simulink model "QCar2_Virtual_Car2"  (R2023a)
settings: Solver=ode1  StartTime=0.0  StopTime=inf  FixedStep=cameraStepSize/10  RelTol=1e-3  EnableMultiTasking=on
PreLoadFcn:
  | QCarSetup
values from neighbouring files (symbols this model uses):
  cameraStepSize = 3e-2    (= 0.03)    [QCarSetup.m]
  path_x = [0.826 0.836 0.846 0.856 0.866 0.876 0.886 0.896 0.906 0.916 0.926 0.936 ... (740 elements, 740x1)]    [SDTS_Paths_6_2023.mat]
  path_x2 = [-0.614 -0.604 -0.594 -0.584 -0.574 -0.564 -0.554 -0.544 -0.534 -0.524 -0.514 -0.504 ... (1090 elements, 1090x1)]    [SDTS_Paths_6_2023.mat]
  path_x3 = [-0.614 -0.603821428571 -0.593642857143 -0.583464285714 -0.573285714286 -0.563107142857 -0.552928571429 -0.54275 -0.532571428571 -0.522392857143 -0.512214285714 -0.502035714286 ... (714 elements, 714x1)]    [SDTS_Paths_6_2023.mat]
  path_x4 = [-0.614 -0.604 -0.594 -0.584 -0.574 -0.564 -0.554 -0.544 -0.534 -0.524 -0.514 -0.504 ... (1761 elements, 1761x1)]    [SDTS_Paths_6_2023.mat]
  path_x5 = [1.436 1.42588571429 1.41577142857 1.40565714286 1.39554285714 1.38542857143 1.37531428571 1.3652 1.35508571429 1.34497142857 1.33485714286 1.32474285714 ... (574 elements, 574x1)]    [SDTS_Paths_6_2023.mat]
  path_x6 = [1.436 1.42588571429 1.41577142857 1.40565714286 1.39554285714 1.38542857143 1.37531428571 1.3652 1.35508571429 1.34497142857 1.33485714286 1.32474285714 ... (1288 elements, 1288x1)]    [SDTS_Paths_6_2023.mat]
  path_y = [-1.0887 -1.0887 -1.0887 -1.0887 -1.0887 -1.0887 -1.0887 -1.0887 -1.0887 -1.0887 -1.0887 -1.0887 ... (740 elements, 740x1)]    [SDTS_Paths_6_2023.mat]
  path_y2 = [-1.0887 -1.0887 -1.0887 -1.0887 -1.0887 -1.0887 -1.0887 -1.0887 -1.0887 -1.0887 -1.0887 -1.0887 ... (1090 elements, 1090x1)]    [SDTS_Paths_6_2023.mat]
  path_y3 = [-1.0887 -1.0887 -1.0887 -1.0887 -1.0887 -1.0887 -1.0887 -1.0887 -1.0887 -1.0887 -1.0887 -1.0887 ... (714 elements, 714x1)]    [SDTS_Paths_6_2023.mat]
  path_y4 = [-1.0887 -1.0887 -1.0887 -1.0887 -1.0887 -1.0887 -1.0887 -1.0887 -1.0887 -1.0887 -1.0887 -1.0887 ... (1761 elements, 1761x1)]    [SDTS_Paths_6_2023.mat]
  path_y5 = [-0.8157 -0.8157 -0.8157 -0.8157 -0.8157 -0.8157 -0.8157 -0.8157 -0.8157 -0.8157 -0.8157 -0.8157 ... (574 elements, 574x1)]    [SDTS_Paths_6_2023.mat]
  path_y6 = [-0.8157 -0.8157 -0.8157 -0.8157 -0.8157 -0.8157 -0.8157 -0.8157 -0.8157 -0.8157 -0.8157 -0.8157 ... (1288 elements, 1288x1)]    [SDTS_Paths_6_2023.mat]
undefined symbols (not defined in the file or in its folder): DiscIntNeverNeededParam, gcbh, height, Host, JPEG, left, qc_get_step_size, top, video_display_show, width
libraries: quarc_library x71, simulink_extras x12, simulink x5
(part 4 of 5)

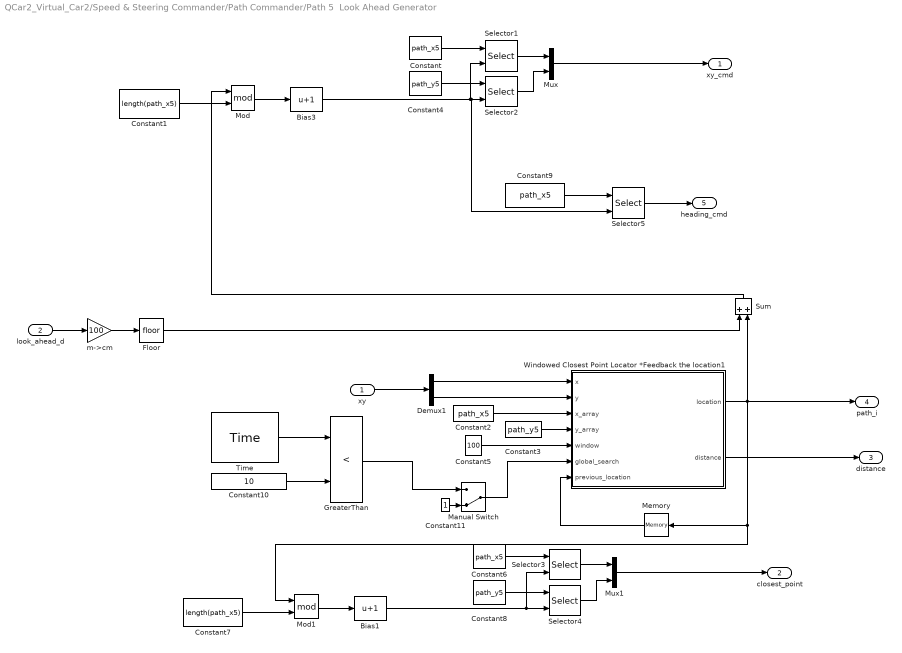
== system QCar2_Virtual_Car2/Speed & Steering Commander/Path Commander/Path 5  Look Ahead Generator ==
  xy : Inport
  look_ahead_d : Inport  Port=2
  Bias1 : Bias  Bias=1  SaturateOnIntegerOverflow=off
  Bias3 : Bias  Bias=1  SaturateOnIntegerOverflow=off
  Constant{,2,6,9} (4 alike) : Constant  Value=path_x5
  Constant1 : Constant  Value=length(path_x5)
  Constant10 : Constant  Value=10
  Constant11 : Constant
  Constant3 : Constant  Value=path_y5
  Constant4 : Constant  Value=path_y5
  Constant5 : Constant  Value=100
  Constant7 : Constant  Value=length(path_x5)
  Constant8 : Constant  Value=path_y5
  Demux1 : Demux  Outputs=2
  Floor : Rounding
  GreaterThan : RelationalOperator  Operator=<  OutDataTypeStr=boolean  RndMeth=Simplest  InputSameDT=off
  Manual Switch : ManualSwitch  CurrentSetting=0
  Memory : Memory  InitialCondition=1  InheritSampleTime=on  LinearizeMemory=on  LinearizeAsDelay=on
  Mod : Math  Operator=mod
  Mod1 : Math  Operator=mod
  Mux : Mux  Inputs=2
  Mux1 : Mux  Inputs=2
  Selector{1..5} (5 alike) : Selector  InputPortWidth=length(path_x5)  IndexOptions=Index vector (port)  Indices=[1 3]  OutputSizes=1
  Sum : Sum
  Time : quarc_library/Sources/Time/Time  time_source=Wall clock  sample_time=qc_get_step_size
  Windowed Closest Point Locator *Feedback the location1 : MATLAB Function  TreatAsAtomicUnit=on
  m->cm : Gain  Gain=100
  xy_cmd : Outport
  closest_point : Outport  Port=2
  distance : Outport  Port=3
  path_i : Outport  Port=4
  heading_cmd : Outport  Port=5
  wires:
  Windowed Closest Point Locator *Feedback the location1/1(location) -> Mod1/1, Memory/1, path_i/1, Sum/2
  Memory/1 -> Windowed Closest Point Locator *Feedback the location1/7(previous_location)
  Constant5/1 -> Windowed Closest Point Locator *Feedback the location1/5(window)
  Selector5/1 -> heading_cmd/1
  Constant9/1 -> Selector5/1
  Bias3/1 -> Selector2/2, Selector5/2, Selector1/2
  Windowed Closest Point Locator *Feedback the location1/2(distance) -> distance/1
  Selector2/1 -> Mux/2
  Mux/1 -> xy_cmd/1
  Constant4/1 -> Selector2/1
  Selector1/1 -> Mux/1
  Constant/1 -> Selector1/1
  Floor/1 -> Sum/1
  m->cm/1 -> Floor/1
  look_ahead_d/1 -> m->cm/1
  xy/1 -> Demux1/1
  Mod/1 -> Bias3/1
  Demux1/2 -> Windowed Closest Point Locator *Feedback the location1/2(y)
  Sum/1 -> Mod/1
  Constant1/1 -> Mod/2
  Constant3/1 -> Windowed Closest Point Locator *Feedback the location1/4(y_array)
  Constant2/1 -> Windowed Closest Point Locator *Feedback the location1/3(x_array)
  Demux1/1 -> Windowed Closest Point Locator *Feedback the location1/1(x)
  Mux1/1 -> closest_point/1
  Mod1/1 -> Bias1/1
  Selector4/1 -> Mux1/2
  Constant7/1 -> Mod1/2
  Selector3/1 -> Mux1/1
  Constant8/1 -> Selector4/1
  Bias1/1 -> Selector3/2, Selector4/2
  Constant6/1 -> Selector3/1
  Time/1 -> GreaterThan/1
  Constant10/1 -> GreaterThan/2
  Manual Switch/1 -> Windowed Closest Point Locator *Feedback the location1/6(global_search)
  Constant11/1 -> Manual Switch/2
  GreaterThan/1 -> Manual Switch/1

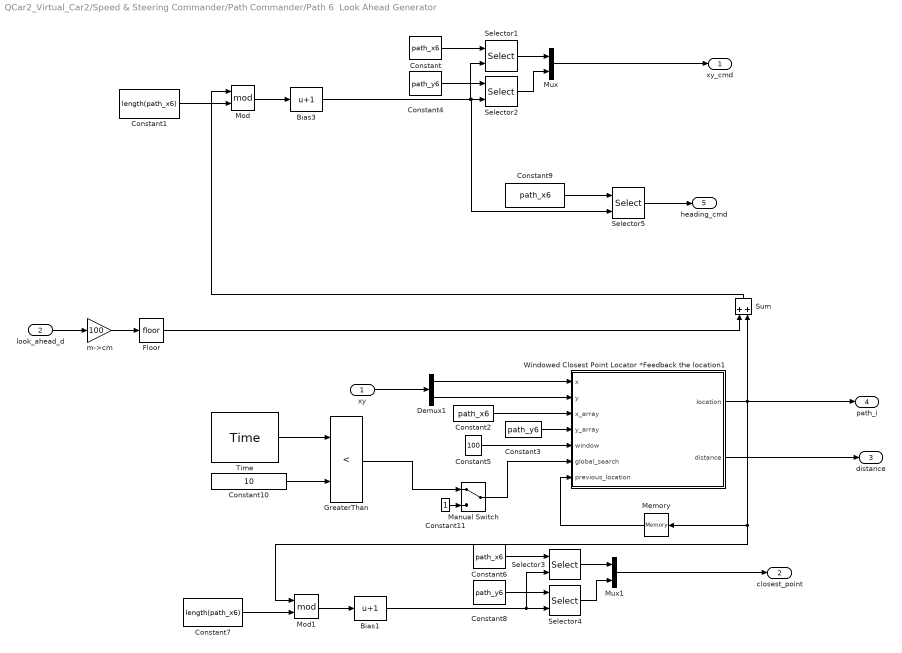
== system QCar2_Virtual_Car2/Speed & Steering Commander/Path Commander/Path 6  Look Ahead Generator ==
  xy : Inport
  look_ahead_d : Inport  Port=2
  Bias1 : Bias  Bias=1  SaturateOnIntegerOverflow=off
  Bias3 : Bias  Bias=1  SaturateOnIntegerOverflow=off
  Constant{,2,6,9} (4 alike) : Constant  Value=path_x6
  Constant1 : Constant  Value=length(path_x6)
  Constant10 : Constant  Value=10
  Constant11 : Constant
  Constant3 : Constant  Value=path_y6
  Constant4 : Constant  Value=path_y6
  Constant5 : Constant  Value=100
  Constant7 : Constant  Value=length(path_x6)
  Constant8 : Constant  Value=path_y6
  Demux1 : Demux  Outputs=2
  Floor : Rounding
  GreaterThan : RelationalOperator  Operator=<  OutDataTypeStr=boolean  RndMeth=Simplest  InputSameDT=off
  Manual Switch : ManualSwitch
  Memory : Memory  InitialCondition=1  InheritSampleTime=on  LinearizeMemory=on  LinearizeAsDelay=on
  Mod : Math  Operator=mod
  Mod1 : Math  Operator=mod
  Mux : Mux  Inputs=2
  Mux1 : Mux  Inputs=2
  Selector{1..5} (5 alike) : Selector  InputPortWidth=length(path_x6)  IndexOptions=Index vector (port)  Indices=[1 3]  OutputSizes=1
  Sum : Sum
  Time : quarc_library/Sources/Time/Time  time_source=Wall clock  sample_time=qc_get_step_size
  Windowed Closest Point Locator *Feedback the location1 : MATLAB Function  TreatAsAtomicUnit=on
  m->cm : Gain  Gain=100
  xy_cmd : Outport
  closest_point : Outport  Port=2
  distance : Outport  Port=3
  path_i : Outport  Port=4
  heading_cmd : Outport  Port=5
  wires:
  GreaterThan/1 -> Manual Switch/1
  Constant11/1 -> Manual Switch/2
  Manual Switch/1 -> Windowed Closest Point Locator *Feedback the location1/6(global_search)
  Constant10/1 -> GreaterThan/2
  Time/1 -> GreaterThan/1
  Constant6/1 -> Selector3/1
  Bias1/1 -> Selector4/2, Selector3/2
  Constant8/1 -> Selector4/1
  Selector3/1 -> Mux1/1
  Constant7/1 -> Mod1/2
  Selector4/1 -> Mux1/2
  Mod1/1 -> Bias1/1
  Mux1/1 -> closest_point/1
  Demux1/1 -> Windowed Closest Point Locator *Feedback the location1/1(x)
  Constant2/1 -> Windowed Closest Point Locator *Feedback the location1/3(x_array)
  Constant3/1 -> Windowed Closest Point Locator *Feedback the location1/4(y_array)
  Constant1/1 -> Mod/2
  Sum/1 -> Mod/1
  Demux1/2 -> Windowed Closest Point Locator *Feedback the location1/2(y)
  Mod/1 -> Bias3/1
  xy/1 -> Demux1/1
  look_ahead_d/1 -> m->cm/1
  m->cm/1 -> Floor/1
  Floor/1 -> Sum/1
  Constant/1 -> Selector1/1
  Selector1/1 -> Mux/1
  Constant4/1 -> Selector2/1
  Mux/1 -> xy_cmd/1
  Selector2/1 -> Mux/2
  Windowed Closest Point Locator *Feedback the location1/2(distance) -> distance/1
  Bias3/1 -> Selector1/2, Selector5/2, Selector2/2
  Constant9/1 -> Selector5/1
  Selector5/1 -> heading_cmd/1
  Constant5/1 -> Windowed Closest Point Locator *Feedback the location1/5(window)
  Memory/1 -> Windowed Closest Point Locator *Feedback the location1/7(previous_location)
  Windowed Closest Point Locator *Feedback the location1/1(location) -> Sum/2, path_i/1, Memory/1, Mod1/1

== system QCar2_Virtual_Car2/Speed & Steering Commander/Traffic Zone 1/Greater Than Threshold ==
  Signal : Inport
  Threshold : Inport  Port=2
  Duration : Inport  Port=3
  Data Type Conversion : DataTypeConversion  SaturateOnIntegerOverflow=off  RndMeth=Floor
  Discrete-Time Integrator : DiscreteIntegrator  Priority=1  ExternalReset=level  SampleTime=qc_get_step_size  ICPrevOutput=DiscIntNeverNeededParam  ICPrevScaledInput=DiscIntNeverNeededParam
  Logical Operator : Logic  Operator=NOT  AllPortsSameDT=off  OutDataTypeStr=boolean
  Relational Operator : RelationalOperator  InputSameDT=off
  Relational Operator1 : RelationalOperator  InputSameDT=off
  elapsed : Outport  VectorParamsAs1DForOutWhenUnconnected=off
  time : Outport  Port=2  VectorParamsAs1DForOutWhenUnconnected=off
  wires:
  Relational Operator1/1 -> elapsed/1
  Duration/1 -> Relational Operator1/2
  Discrete-Time Integrator/1 -> time/1, Relational Operator1/1
  Logical Operator/1 -> Discrete-Time Integrator/2
  Relational Operator/1 -> Logical Operator/1, Data Type Conversion/1
  Threshold/1 -> Relational Operator/2
  Signal/1 -> Relational Operator/1
  Data Type Conversion/1 -> Discrete-Time Integrator/1

== system QCar2_Virtual_Car2/Speed & Steering Commander/Traffic Zone 1/Less Than Threshold ==
  Signal : Inport
  Threshold : Inport  Port=2
  Duration : Inport  Port=3
  Data Type Conversion : DataTypeConversion  SaturateOnIntegerOverflow=off  RndMeth=Floor
  Discrete-Time Integrator : DiscreteIntegrator  Priority=1  ExternalReset=level  SampleTime=qc_get_step_size  ICPrevOutput=DiscIntNeverNeededParam  ICPrevScaledInput=DiscIntNeverNeededParam
  Logical Operator : Logic  Operator=NOT  AllPortsSameDT=off  OutDataTypeStr=boolean
  Relational Operator : RelationalOperator  Operator=<  InputSameDT=off
  Relational Operator1 : RelationalOperator  InputSameDT=off
  elapsed : Outport  VectorParamsAs1DForOutWhenUnconnected=off
  time : Outport  Port=2  VectorParamsAs1DForOutWhenUnconnected=off
  wires:
  Data Type Conversion/1 -> Discrete-Time Integrator/1
  Signal/1 -> Relational Operator/1
  Threshold/1 -> Relational Operator/2
  Relational Operator/1 -> Data Type Conversion/1, Logical Operator/1
  Logical Operator/1 -> Discrete-Time Integrator/2
  Discrete-Time Integrator/1 -> Relational Operator1/1, time/1
  Duration/1 -> Relational Operator1/2
  Relational Operator1/1 -> elapsed/1

== system QCar2_Virtual_Car2/Speed & Steering Commander/Traffic Zone 2/Greater Than Threshold ==
  Signal : Inport
  Threshold : Inport  Port=2
  Duration : Inport  Port=3
  Data Type Conversion : DataTypeConversion  SaturateOnIntegerOverflow=off  RndMeth=Floor
  Discrete-Time Integrator : DiscreteIntegrator  Priority=1  ExternalReset=level  SampleTime=qc_get_step_size  ICPrevOutput=DiscIntNeverNeededParam  ICPrevScaledInput=DiscIntNeverNeededParam
  Logical Operator : Logic  Operator=NOT  AllPortsSameDT=off  OutDataTypeStr=boolean
  Relational Operator : RelationalOperator  InputSameDT=off
  Relational Operator1 : RelationalOperator  InputSameDT=off
  elapsed : Outport  VectorParamsAs1DForOutWhenUnconnected=off
  time : Outport  Port=2  VectorParamsAs1DForOutWhenUnconnected=off
  wires:
  Data Type Conversion/1 -> Discrete-Time Integrator/1
  Signal/1 -> Relational Operator/1
  Threshold/1 -> Relational Operator/2
  Relational Operator/1 -> Data Type Conversion/1, Logical Operator/1
  Logical Operator/1 -> Discrete-Time Integrator/2
  Discrete-Time Integrator/1 -> Relational Operator1/1, time/1
  Duration/1 -> Relational Operator1/2
  Relational Operator1/1 -> elapsed/1

== system QCar2_Virtual_Car2/Speed & Steering Commander/Traffic Zone 2/Less Than Threshold ==
  Signal : Inport
  Threshold : Inport  Port=2
  Duration : Inport  Port=3
  Data Type Conversion : DataTypeConversion  SaturateOnIntegerOverflow=off  RndMeth=Floor
  Discrete-Time Integrator : DiscreteIntegrator  Priority=1  ExternalReset=level  SampleTime=qc_get_step_size  ICPrevOutput=DiscIntNeverNeededParam  ICPrevScaledInput=DiscIntNeverNeededParam
  Logical Operator : Logic  Operator=NOT  AllPortsSameDT=off  OutDataTypeStr=boolean
  Relational Operator : RelationalOperator  Operator=<  InputSameDT=off
  Relational Operator1 : RelationalOperator  InputSameDT=off
  elapsed : Outport  VectorParamsAs1DForOutWhenUnconnected=off
  time : Outport  Port=2  VectorParamsAs1DForOutWhenUnconnected=off
  wires:
  Relational Operator1/1 -> elapsed/1
  Duration/1 -> Relational Operator1/2
  Discrete-Time Integrator/1 -> time/1, Relational Operator1/1
  Logical Operator/1 -> Discrete-Time Integrator/2
  Relational Operator/1 -> Logical Operator/1, Data Type Conversion/1
  Threshold/1 -> Relational Operator/2
  Signal/1 -> Relational Operator/1
  Data Type Conversion/1 -> Discrete-Time Integrator/1

== system QCar2_Virtual_Car2/Cameras/CSI Camera/Extract Center and Slope/Angle Check ==
  score : Inport
  Angle In : Inport  Port=2
  score threshold : Inport  Port=3
  IsNaN : RelationalOperator  Operator=isNaN  OutDataTypeStr=boolean  RndMeth=Simplest  InputSameDT=off
  Less Than : RelationalOperator  Operator=<  OutDataTypeStr=boolean  RndMeth=Simplest  InputSameDT=off
  MATLAB Function1 : MATLAB Function  TreatAsAtomicUnit=on
  Memory : Memory  InheritSampleTime=on  LinearizeMemory=on  LinearizeAsDelay=on
  OR : Logic  Operator=OR  IconShape=distinctive  AllPortsSameDT=off  OutDataTypeStr=boolean
  Angle Out : Outport  VectorParamsAs1DForOutWhenUnconnected=off
  wires:
  IsNaN/1 -> OR/1
  OR/1 -> MATLAB Function1/2(is_nan)
  Less Than/1 -> OR/2
  score/1 -> Less Than/1
  score threshold/1 -> Less Than/2
  MATLAB Function1/1(output) -> Angle Out/1, Memory/1
  Angle In/1 -> MATLAB Function1/1(input), IsNaN/1
  Memory/1 -> MATLAB Function1/3(prev_output)

== system QCar2_Virtual_Car2/Cameras/CSI Camera/Extract Center and Slope/Center Check ==
  score : Inport
  Center : Inport  Port=2
  score threshold : Inport  Port=3
  IsNaN : RelationalOperator  Operator=isNaN  OutDataTypeStr=boolean  RndMeth=Simplest  InputSameDT=off
  Less Than : RelationalOperator  Operator=<  OutDataTypeStr=boolean  RndMeth=Simplest  InputSameDT=off
  MATLAB Function1 : MATLAB Function  TreatAsAtomicUnit=on
  Memory : Memory  InitialCondition=640/2  InheritSampleTime=on  LinearizeMemory=on  LinearizeAsDelay=on
  OR : Logic  Operator=OR  IconShape=distinctive  AllPortsSameDT=off  OutDataTypeStr=boolean
  Center Out : Outport  VectorParamsAs1DForOutWhenUnconnected=off
  wires:
  score threshold/1 -> Less Than/2
  Less Than/1 -> OR/2
  score/1 -> Less Than/1
  IsNaN/1 -> OR/1
  OR/1 -> MATLAB Function1/2(is_nan)
  Memory/1 -> MATLAB Function1/3(prev_output)
  Center/1 -> IsNaN/1, MATLAB Function1/1(input)
  MATLAB Function1/1(output) -> Memory/1, Center Out/1

== system QCar2_Virtual_Car2/QCar/Virtual QCar/LED Logic/Greater Than Threshold1 ==
  Signal : Inport
  Threshold : Inport  Port=2
  Duration : Inport  Port=3
  Data Type Conversion : DataTypeConversion  SaturateOnIntegerOverflow=off  RndMeth=Floor
  Discrete-Time Integrator : DiscreteIntegrator  Priority=1  ExternalReset=level  SampleTime=qc_get_step_size  ICPrevOutput=DiscIntNeverNeededParam  ICPrevScaledInput=DiscIntNeverNeededParam
  Logical Operator : Logic  Operator=NOT  AllPortsSameDT=off  OutDataTypeStr=boolean
  Relational Operator : RelationalOperator  InputSameDT=off
  Relational Operator1 : RelationalOperator  InputSameDT=off
  elapsed : Outport  VectorParamsAs1DForOutWhenUnconnected=off
  time : Outport  Port=2  VectorParamsAs1DForOutWhenUnconnected=off
  wires:
  Data Type Conversion/1 -> Discrete-Time Integrator/1
  Signal/1 -> Relational Operator/1
  Threshold/1 -> Relational Operator/2
  Relational Operator/1 -> Data Type Conversion/1, Logical Operator/1
  Logical Operator/1 -> Discrete-Time Integrator/2
  Discrete-Time Integrator/1 -> Relational Operator1/1, time/1
  Duration/1 -> Relational Operator1/2
  Relational Operator1/1 -> elapsed/1

== system QCar2_Virtual_Car2/QCar/Virtual QCar/LED Logic/Left Threshold ==
  Signal : Inport
  Threshold : Inport  Port=2
  Duration : Inport  Port=3
  Data Type Conversion : DataTypeConversion  SaturateOnIntegerOverflow=off  RndMeth=Floor
  Discrete-Time Integrator : DiscreteIntegrator  Priority=1  ExternalReset=level  SampleTime=qc_get_step_size  ICPrevOutput=DiscIntNeverNeededParam  ICPrevScaledInput=DiscIntNeverNeededParam
  Logical Operator : Logic  Operator=NOT  AllPortsSameDT=off  OutDataTypeStr=boolean
  Relational Operator : RelationalOperator  InputSameDT=off
  Relational Operator1 : RelationalOperator  InputSameDT=off
  elapsed : Outport  VectorParamsAs1DForOutWhenUnconnected=off
  time : Outport  Port=2  VectorParamsAs1DForOutWhenUnconnected=off
  wires:
  Data Type Conversion/1 -> Discrete-Time Integrator/1
  Signal/1 -> Relational Operator/1
  Threshold/1 -> Relational Operator/2
  Relational Operator/1 -> Data Type Conversion/1, Logical Operator/1
  Logical Operator/1 -> Discrete-Time Integrator/2
  Discrete-Time Integrator/1 -> Relational Operator1/1, time/1
  Duration/1 -> Relational Operator1/2
  Relational Operator1/1 -> elapsed/1

== system QCar2_Virtual_Car2/QCar/Virtual QCar/LED Logic/Less Than Threshold1 ==
  Signal : Inport
  Threshold : Inport  Port=2
  Duration : Inport  Port=3
  Data Type Conversion : DataTypeConversion  SaturateOnIntegerOverflow=off  RndMeth=Floor
  Discrete-Time Integrator : DiscreteIntegrator  Priority=1  ExternalReset=level  SampleTime=qc_get_step_size  ICPrevOutput=DiscIntNeverNeededParam  ICPrevScaledInput=DiscIntNeverNeededParam
  Logical Operator : Logic  Operator=NOT  AllPortsSameDT=off  OutDataTypeStr=boolean
  Relational Operator : RelationalOperator  Operator=<  InputSameDT=off
  Relational Operator1 : RelationalOperator  InputSameDT=off
  elapsed : Outport  VectorParamsAs1DForOutWhenUnconnected=off
  time : Outport  Port=2  VectorParamsAs1DForOutWhenUnconnected=off
  wires:
  Relational Operator1/1 -> elapsed/1
  Duration/1 -> Relational Operator1/2
  Discrete-Time Integrator/1 -> time/1, Relational Operator1/1
  Logical Operator/1 -> Discrete-Time Integrator/2
  Relational Operator/1 -> Logical Operator/1, Data Type Conversion/1
  Threshold/1 -> Relational Operator/2
  Signal/1 -> Relational Operator/1
  Data Type Conversion/1 -> Discrete-Time Integrator/1

== system QCar2_Virtual_Car2/QCar/Virtual QCar/LED Logic/Less Than Threshold2 ==
  Signal : Inport
  Threshold : Inport  Port=2
  Duration : Inport  Port=3
  Data Type Conversion : DataTypeConversion  SaturateOnIntegerOverflow=off  RndMeth=Floor
  Discrete-Time Integrator : DiscreteIntegrator  Priority=1  ExternalReset=level  SampleTime=qc_get_step_size  ICPrevOutput=DiscIntNeverNeededParam  ICPrevScaledInput=DiscIntNeverNeededParam
  Logical Operator : Logic  Operator=NOT  AllPortsSameDT=off  OutDataTypeStr=boolean
  Relational Operator : RelationalOperator  Operator=<  InputSameDT=off
  Relational Operator1 : RelationalOperator  InputSameDT=off
  elapsed : Outport  VectorParamsAs1DForOutWhenUnconnected=off
  time : Outport  Port=2  VectorParamsAs1DForOutWhenUnconnected=off
  wires:
  Data Type Conversion/1 -> Discrete-Time Integrator/1
  Signal/1 -> Relational Operator/1
  Threshold/1 -> Relational Operator/2
  Relational Operator/1 -> Data Type Conversion/1, Logical Operator/1
  Logical Operator/1 -> Discrete-Time Integrator/2
  Discrete-Time Integrator/1 -> Relational Operator1/1, time/1
  Duration/1 -> Relational Operator1/2
  Relational Operator1/1 -> elapsed/1

== system QCar2_Virtual_Car2/QCar/Virtual QCar/LED Logic/Less Than Threshold3 ==
  Signal : Inport
  Threshold : Inport  Port=2
  Duration : Inport  Port=3
  Data Type Conversion : DataTypeConversion  SaturateOnIntegerOverflow=off  RndMeth=Floor
  Discrete-Time Integrator : DiscreteIntegrator  Priority=1  ExternalReset=level  SampleTime=qc_get_step_size  ICPrevOutput=DiscIntNeverNeededParam  ICPrevScaledInput=DiscIntNeverNeededParam
  Logical Operator : Logic  Operator=NOT  AllPortsSameDT=off  OutDataTypeStr=boolean
  Relational Operator : RelationalOperator  Operator=<  InputSameDT=off
  Relational Operator1 : RelationalOperator  InputSameDT=off
  elapsed : Outport  VectorParamsAs1DForOutWhenUnconnected=off
  time : Outport  Port=2  VectorParamsAs1DForOutWhenUnconnected=off
  wires:
  Relational Operator1/1 -> elapsed/1
  Duration/1 -> Relational Operator1/2
  Discrete-Time Integrator/1 -> time/1, Relational Operator1/1
  Logical Operator/1 -> Discrete-Time Integrator/2
  Relational Operator/1 -> Logical Operator/1, Data Type Conversion/1
  Threshold/1 -> Relational Operator/2
  Signal/1 -> Relational Operator/1
  Data Type Conversion/1 -> Discrete-Time Integrator/1

== system QCar2_Virtual_Car2/QCar/Virtual QCar/LED Logic/Right Threshold ==
  Signal : Inport
  Threshold : Inport  Port=2
  Duration : Inport  Port=3
  Data Type Conversion : DataTypeConversion  SaturateOnIntegerOverflow=off  RndMeth=Floor
  Discrete-Time Integrator : DiscreteIntegrator  Priority=1  ExternalReset=level  SampleTime=qc_get_step_size  ICPrevOutput=DiscIntNeverNeededParam  ICPrevScaledInput=DiscIntNeverNeededParam
  Logical Operator : Logic  Operator=NOT  AllPortsSameDT=off  OutDataTypeStr=boolean
  Relational Operator : RelationalOperator  Operator=<  InputSameDT=off
  Relational Operator1 : RelationalOperator  InputSameDT=off
  elapsed : Outport  VectorParamsAs1DForOutWhenUnconnected=off
  time : Outport  Port=2  VectorParamsAs1DForOutWhenUnconnected=off
  wires:
  Data Type Conversion/1 -> Discrete-Time Integrator/1
  Signal/1 -> Relational Operator/1
  Threshold/1 -> Relational Operator/2
  Relational Operator/1 -> Data Type Conversion/1, Logical Operator/1
  Logical Operator/1 -> Discrete-Time Integrator/2
  Discrete-Time Integrator/1 -> Relational Operator1/1, time/1
  Duration/1 -> Relational Operator1/2
  Relational Operator1/1 -> elapsed/1

== matlab function QCar2_Virtual_Car2/Speed & Steering Commander/Traffic Zone 2/MATLAB Function2 ==
  data: Previous_State input; Speed_In input; Speed_Multi input; In_Zone input; Traffic_State output; Speed_Out output; Traffic_Light input
function [Traffic_State, Speed_Out]  = Traffic_Controller (Previous_State, Speed_In, Speed_Multi, In_Zone, Traffic_Light)
%#codegen
Traffic_State = Previous_State;
Speed_Out = Speed_In;

switch Traffic_State
    % Case 1 - Normal - either not in zone or green light, Case 2 - red
    % light and in zone
    
    case 1
        % Green light or not in zone
        Speed_Out = Speed_In;
        if (Traffic_Light == 0) && (In_Zone == 1)
            % Caught in the traffic controller's web!
            Traffic_State = 2;
        end
        
    case 2
        % Red light state
        Speed_Out = Speed_In * Speed_Multi;
        
        if (Traffic_Light == 1)
            % Green Light
            Traffic_State = 1;
        end
        
end
end

== matlab function QCar2_Virtual_Car2/QCar/To//From Simulation/Receive Fcn ==
  data: Receive input size=800000; RequestServerUpdate output; New input; Location output; Rotation output; BumpForward output; BumpRear output; EnvironmentReset output; LidarDist output; LidarAngle output; NewCSIRight output; ImageCSIRight output size=100000; NewCSIRear output; ImageCSIRear output size=100000; NewCSILeft output; ImageCSILeft output size=100000; NewCSIFront output; ImageCSIFront output size=100000; NewRGB output; ImageRGB output size=100000; NewDepth output; ImageDepth output size=100000; Debug output
function [RequestServerUpdate, Location, Rotation, BumpForward, BumpRear, EnvironmentReset, LidarDist, LidarAngle, ...
    NewCSIRight, ImageCSIRight, ...
    NewCSIRear, ImageCSIRear, ...
    NewCSILeft, ImageCSILeft, ...
    NewCSIFront, ImageCSIFront, ...
    NewRGB, ImageRGB, ...
    NewDepth, ImageDepth, ...
    Debug]  = QCar2ApplicationWorkspaceDecodeDataPacket(Receive, New)

%% Setup

LIDAR_SAMPLES = 384;
LIDAR_RANGE = 80;

persistent iLocation;
persistent iRotation;
persistent iBumpForward;
persistent iBumpRear;
persistent iLidarDist;
persistent iLidarAngle;

if isempty(iLocation)
    iLocation = [single(0); single(0); single(0)];
    iRotation = [single(0); single(0); single(0)];
    iBumpForward = uint8(0);
    iBumpRear = uint8(0);
    iLidarAngle = zeros(1,LIDAR_SAMPLES);   
    iLidarDist = zeros(1,LIDAR_SAMPLES);      
end

% Need to assign outputs here even though they are reassigned at the end
% since matlab can't determine the signal widths
Location = [single(0); single(0); single(0)];
Rotation = [single(0); single(0); single(0)];
BumpForward = uint8(0);
BumpRear = uint8(0);
EnvironmentReset = 0;

LidarAngle = zeros(1,LIDAR_SAMPLES);
LidarDist = zeros(1,LIDAR_SAMPLES);

ImageCSIRight = uint8([]);
NewCSIRight = 0;
ImageCSIRear = uint8([]);
NewCSIRear = 0;
ImageCSILeft = uint8([]);
NewCSILeft = 0;
ImageCSIFront = uint8([]);
NewCSIFront = 0;
ImageRGB = uint8([]);
NewRGB = 0;
ImageDepth = uint8([]);
NewDepth = 0;


RequestServerUpdate = uint8(0);
PacketSize = length(Receive);

Debug = int32(0);

% Packet > 0, new data, and magic number in first index
if ((PacketSize > 0) && (New == 1) && (Receive(1) == uint8(123)))
    
    %skip magic number
    Index = int32(2);
    
    while(Index <= PacketSize)
       
        %% Get container details
        ContainerSize = typecast(uint8(flip(Receive(Index:Index+3))), 'int32');
        DeviceID = typecast(uint8(flip(Receive(Index+4:Index+7))), 'int32');
        DeviceNum = typecast(uint8(flip(Receive(Index+8:Index+11))), 'int32');
        DeviceFunction = uint8(Receive(Index+12));
        PayloadStart = Index+13;
        PayloadEnd = Index+ContainerSize-1;
        
        %% Pass container to appropriate decoding function
        if (DeviceID == 161) %is this a QCar 2 container?
            
            if (DeviceFunction == 11) %UE4 State Response
                [iLocation, iRotation, iBumpForward, iBumpRear] = QCar2DecodeVelocityStateContainer(Receive, PayloadStart);
                RequestServerUpdate = uint8(11);
            elseif (DeviceFunction == 101) % Pull out RGB payload for external processing
                CameraNum = typecast(uint8(flip(Receive(PayloadStart:PayloadStart+3))), 'int32');
                ImageSize = typecast(uint8(flip(Receive(PayloadStart+4:PayloadStart+7))), 'int32');
                
                if CameraNum == 0
                    ImageCSIRight = Receive(PayloadStart+8:PayloadEnd);
                    NewCSIRight = 1;
                    
                elseif CameraNum == 1
                    ImageCSIRear = Receive(PayloadStart+8:PayloadEnd);
                    NewCSIRear = 1;
                    
                elseif CameraNum == 2
                    ImageCSILeft = Receive(PayloadStart+8:PayloadEnd);
                    NewCSILeft = 1;
                    
                elseif CameraNum == 3
                    ImageCSIFront = Receive(PayloadStart+8:PayloadEnd);
                    NewCSIFront = 1;
                    
                elseif CameraNum == 4
                    ImageRGB = Receive(PayloadStart+8:PayloadEnd);
                    NewRGB = 1;
                    
                elseif CameraNum == 5
                    ImageDepth = Receive(PayloadStart+8:PayloadEnd);
                    NewDepth = 1;
                end
                RequestServerUpdate = uint8(1);

            elseif (DeviceFunction == 111) % Process LIDAR
                [iLidarAngle, iLidarDist] = QCar2DecodeLidarContainer(Receive, PayloadStart, LIDAR_SAMPLES, LIDAR_RANGE);
                RequestServerUpdate = uint8(1);                
            end
        elseif (DeviceID == 1001) %Simulink notification
            if (DeviceFunction == 200) %Reset button
                EnvironmentReset = 1;
            end
            


        end
       
        
        %% Process next container if any data is left.
        Index = Index+ContainerSize;
    end


end

Location = iLocation;
Rotation = iRotation;
BumpForward = iBumpForward;
BumpRear = iBumpRear;
LidarDist = iLidarDist;
LidarAngle = iLidarAngle;

== matlab function QCar2_Virtual_Car2/Speed & Steering Commander/Adaptive Cruise Control/MATLAB Function ==
  data: obstacle_distance input; speed_cmd output; stop_distance input; nominal_tracking_distance input; nominal_speed input
function speed_cmd = adaptive_cruise_control(obstacle_distance, stop_distance, nominal_tracking_distance, nominal_speed)

speed_cmd = nominal_speed;

if obstacle_distance < stop_distance
    speed_cmd = sat(nominal_speed,0,-1);
    
elseif obstacle_distance < nominal_tracking_distance
    speed_cmd = nominal_speed/(nominal_tracking_distance-stop_distance)*obstacle_distance - nominal_speed/(nominal_tracking_distance-stop_distance)*stop_distance;
end

function output = sat (input, max,min)
if input > max
    output = max;
elseif input < min
    output = min;
else
    output = input;
end

== matlab function QCar2_Virtual_Car2/Speed & Steering Commander/LiDAR Steering/Steering Commander ==
  data: steering output; aoa input
function steering  = steering_command(aoa)
steering = aoa;
if aoa < -pi
    steering = aoa+2*pi;
elseif aoa > pi
    steering = aoa-2*pi;
else
    steering = aoa;
end
end

== matlab function QCar2_Virtual_Car2/Cameras/CSI Camera/Extract Center and Slope/Center Check/MATLAB Function1 ==
  data: input input; output output; is_nan input; prev_output input
function output = fcn(input, is_nan, prev_output)
if is_nan == 1
    output = prev_output;
else
    output = input;
end

== matlab function QCar2_Virtual_Car2/QCar/To//From Simulation/Transmit Fcn ==
  settings: updateMethod=DISCRETE  sampleTime=qc_get_step_size
  data: Packet output size=65537; ServerState input; SendUpdate input; Enable output; DeviceNumber input; Forward_And_Steering input; Lights input; EnableCameras input; LEDStrip input; LEDStripNew input; EnableLIDAR input
function [Packet,Enable] = QCar2ApplicationWorkspaceMakePacketData(ServerState, SendUpdate, DeviceNumber, Forward_And_Steering, Lights, EnableCameras, LEDStrip, LEDStripNew, EnableLIDAR) 

% Be sure to set the maximum signal size of the variable size Packet port 
% in Simulink->Edit Data of the editor window.  Size should be 65537 or
% larger to ensure that the stream server generates a 4 byte packet size.

%% Setup
persistent LastServerState;
persistent LastLEDStrip;

if isempty(LastServerState)
    LastServerState = uint8(0);

    % Initialize with -1 to ensure it will always send the first update.
    LastLEDStrip = -1*ones(3,33);
end

Enable = 0;
Packet = uint8([]);


%% Send new State Container or On connection
% Previous state processed, send a new one
if (SendUpdate) || ((ServerState == 2) && (LastServerState ~= 2))
    Packet = QCar2MakeCommandVelocityStateContainer(DeviceNumber, Forward_And_Steering, Lights);
    
    for (index = 1:6)
        if (EnableCameras(index))
            Packet = [Packet; QCar2MakeCameraRequestContainer(DeviceNumber, index-1)];
        end
    end

    if (LEDStripNew)
        % This is an expensive operation so only send this if it has
        % changed.
        if ~all(all(LastLEDStrip == LEDStrip))
            LastLEDStrip = LEDStrip;
            Brightness = 10;
            Packet = [Packet; QCar2MakeSetLEDStripContainer(DeviceNumber, LEDStrip, Brightness)];
        end
    end

    if (EnableLIDAR)
        Packet = [Packet; QCar2MakeLidarRequestContainer(DeviceNumber)];
    end
end

%% Transmit
% If we have data to send, enable the transmit
PacketLength = length(Packet);

if (PacketLength > 0)
    % Add magic byte.  This is just for error handling and isn't typically
    % required in simulink, but useful in lower-level languages like Python
    Packet = [uint8(123); Packet];
    
    Enable = 1; 
end


LastServerState = ServerState;

== matlab function QCar2_Virtual_Car2/Speed & Steering Commander/MATLAB Function2 ==
  data: Previous_State input; Stop_Sign input; Sign_Time input; No_Sign_Time input; Sign_State output; Speed_Multiplier output; Step_size input; Previous_Timer input; Timer output
function [Sign_State, Speed_Multiplier, Timer]  = NN_Decipher (Previous_State, Stop_Sign, Sign_Time, No_Sign_Time, Step_size,Previous_Timer)
%#codegen
Sign_State = Previous_State;
Timer = Previous_Timer + Step_size;
Speed_Multiplier = 1;

switch Sign_State
    % Case 1 - No Sign, Case 2 - Stop Sign, Case 3 - Slow Sign
    
    case 1
        % No Signs Found
        Speed_Multiplier = 1;
        if (Timer > No_Sign_Time)
            % Stay in the No Sign state for a while each time
            if (Stop_Sign == 1)
                Sign_State = 2;
                Timer = 0;
%             elseif  (Slow_Sign == 1)
%                 Sign_State = 3;
%                 Timer = 0;
            end
        end
        
    case 2
        % Stop Sign State
        Speed_Multiplier = 0;
        %         Signs_Out = [0 Signs_In(2) Slow_Sign 1 Signs_In(5)];
        Signs_Out = [0 0 0 1 0];
        if (Timer > Sign_Time)
            % Goto Normal State
            Sign_State = 1;
            Timer = 0;
        end
              
end
end

== matlab function QCar2_Virtual_Car2/Speed & Steering Commander/Path Commander/Path 1  Look Ahead Generator/Windowed Closest Point Locator *Feedback the location1 ==
  data: x input; location output; y input; x_array input; y_array input; window input; global_search input; distance output; previous_location input
function [location,distance] = find_closest_window_point(x,y,x_array,y_array, window, global_search, previous_location)
distance = 1e6;
location = previous_location;
array_length = length (x_array);

if (global_search == 1)
    
    %Search the whole array (usually at startup)
    for i =1:array_length
        d = (x-x_array(i))^2 + (y-y_array(i))^2;
        if d < distance
            distance = d;
            location = i;
        end
    end
    
else
    
    if (location + window) > array_length
        %We need to wrap from the end
        % loop one - end of array:
        for i = (location-window):array_length
            d = (x-x_array(i))^2 + (y-y_array(i))^2;
            if d < distance
                distance = d;
                location = i;
            end
        end
        % loop two - start of array:
        for i = 1:(location+window-array_length)
            d = (x-x_array(i))^2 + (y-y_array(i))^2;
            if d < distance
                distance = d;
                location = i;
            end
        end
        
    elseif (location-window) < 1
        %We need to wrap from the beginning
        % loop one - end of array:
        for i = (array_length+location-window):array_length
            d = (x-x_array(i))^2 + (y-y_array(i))^2;
            if d < distance
                distance = d;
                location = i;
            end
        end
        % loop two - start of array:
        for i = 1:(location+window)
            d = (x-x_array(i))^2 + (y-y_array(i))^2;
            if d < distance
                distance = d;
                location = i;
            end
        end
        
    else
        %no need to wrap
        for i = (location-window):(location+window)
            d = (x-x_array(i))^2 + (y-y_array(i))^2;
            if d < distance
                distance = d;
                location = i;
            end
        end
    end
    
end
distance = sqrt(distance);
end

== matlab function QCar2_Virtual_Car2/Speed & Steering Commander/Path Commander/Path 2  Look Ahead Generator/Windowed Closest Point Locator *Feedback the location1 ==
  data: x input; location output; y input; x_array input; y_array input; window input; global_search input; distance output; previous_location input
function [location,distance] = find_closest_window_point(x,y,x_array,y_array, window, global_search, previous_location)
distance = 1e6;
location = previous_location;
array_length = length (x_array);

if (global_search == 1)
    
    %Search the whole array (usually at startup)
    for i =1:array_length
        d = (x-x_array(i))^2 + (y-y_array(i))^2;
        if d < distance
            distance = d;
            location = i;
        end
    end
    
else
    
    if (location + window) > array_length
        %We need to wrap from the end
        % loop one - end of array:
        for i = (location-window):array_length
            d = (x-x_array(i))^2 + (y-y_array(i))^2;
            if d < distance
                distance = d;
                location = i;
            end
        end
        % loop two - start of array:
        for i = 1:(location+window-array_length)
            d = (x-x_array(i))^2 + (y-y_array(i))^2;
            if d < distance
                distance = d;
                location = i;
            end
        end
        
    elseif (location-window) < 1
        %We need to wrap from the beginning
        % loop one - end of array:
        for i = (array_length+location-window):array_length
            d = (x-x_array(i))^2 + (y-y_array(i))^2;
            if d < distance
                distance = d;
                location = i;
            end
        end
        % loop two - start of array:
        for i = 1:(location+window)
            d = (x-x_array(i))^2 + (y-y_array(i))^2;
            if d < distance
                distance = d;
                location = i;
            end
        end
        
    else
        %no need to wrap
        for i = (location-window):(location+window)
            d = (x-x_array(i))^2 + (y-y_array(i))^2;
            if d < distance
                distance = d;
                location = i;
            end
        end
    end
    
end
distance = sqrt(distance);
end

== matlab function QCar2_Virtual_Car2/Speed & Steering Commander/Path Commander/Path 3  Look Ahead Generator/Windowed Closest Point Locator *Feedback the location1 ==
  data: x input; location output; y input; x_array input; y_array input; window input; global_search input; distance output; previous_location input
function [location,distance] = find_closest_window_point(x,y,x_array,y_array, window, global_search, previous_location)
distance = 1e6;
location = previous_location;
array_length = length (x_array);

if (global_search == 1)
    
    %Search the whole array (usually at startup)
    for i =1:array_length
        d = (x-x_array(i))^2 + (y-y_array(i))^2;
        if d < distance
            distance = d;
            location = i;
        end
    end
    
else
    
    if (location + window) > array_length
        %We need to wrap from the end
        % loop one - end of array:
        for i = (location-window):array_length
            d = (x-x_array(i))^2 + (y-y_array(i))^2;
            if d < distance
                distance = d;
                location = i;
            end
        end
        % loop two - start of array:
        for i = 1:(location+window-array_length)
            d = (x-x_array(i))^2 + (y-y_array(i))^2;
            if d < distance
                distance = d;
                location = i;
            end
        end
        
    elseif (location-window) < 1
        %We need to wrap from the beginning
        % loop one - end of array:
        for i = (array_length+location-window):array_length
            d = (x-x_array(i))^2 + (y-y_array(i))^2;
            if d < distance
                distance = d;
                location = i;
            end
        end
        % loop two - start of array:
        for i = 1:(location+window)
            d = (x-x_array(i))^2 + (y-y_array(i))^2;
            if d < distance
                distance = d;
                location = i;
            end
        end
        
    else
        %no need to wrap
        for i = (location-window):(location+window)
            d = (x-x_array(i))^2 + (y-y_array(i))^2;
            if d < distance
                distance = d;
                location = i;
            end
        end
    end
    
end
distance = sqrt(distance);
end

== matlab function QCar2_Virtual_Car2/Speed & Steering Commander/Path Commander/Path 4  Look Ahead Generator/Windowed Closest Point Locator *Feedback the location1 ==
  data: x input; location output; y input; x_array input; y_array input; window input; global_search input; distance output; previous_location input
function [location,distance] = find_closest_window_point(x,y,x_array,y_array, window, global_search, previous_location)
distance = 1e6;
location = previous_location;
array_length = length (x_array);

if (global_search == 1)
    
    %Search the whole array (usually at startup)
    for i =1:array_length
        d = (x-x_array(i))^2 + (y-y_array(i))^2;
        if d < distance
            distance = d;
            location = i;
        end
    end
    
else
    
    if (location + window) > array_length
        %We need to wrap from the end
        % loop one - end of array:
        for i = (location-window):array_length
            d = (x-x_array(i))^2 + (y-y_array(i))^2;
            if d < distance
                distance = d;
                location = i;
            end
        end
        % loop two - start of array:
        for i = 1:(location+window-array_length)
            d = (x-x_array(i))^2 + (y-y_array(i))^2;
            if d < distance
                distance = d;
                location = i;
            end
        end
        
    elseif (location-window) < 1
        %We need to wrap from the beginning
        % loop one - end of array:
        for i = (array_length+location-window):array_length
            d = (x-x_array(i))^2 + (y-y_array(i))^2;
            if d < distance
                distance = d;
                location = i;
            end
        end
        % loop two - start of array:
        for i = 1:(location+window)
            d = (x-x_array(i))^2 + (y-y_array(i))^2;
            if d < distance
                distance = d;
                location = i;
            end
        end
        
    else
        %no need to wrap
        for i = (location-window):(location+window)
            d = (x-x_array(i))^2 + (y-y_array(i))^2;
            if d < distance
                distance = d;
                location = i;
            end
        end
    end
    
end
distance = sqrt(distance);
end

== matlab function QCar2_Virtual_Car2/Speed & Steering Commander/Path Commander/Path 5  Look Ahead Generator/Windowed Closest Point Locator *Feedback the location1 ==
  data: x input; location output; y input; x_array input; y_array input; window input; global_search input; distance output; previous_location input
function [location,distance] = find_closest_window_point(x,y,x_array,y_array, window, global_search, previous_location)
distance = 1e6;
location = previous_location;
array_length = length (x_array);

if (global_search == 1)
    
    %Search the whole array (usually at startup)
    for i =1:array_length
        d = (x-x_array(i))^2 + (y-y_array(i))^2;
        if d < distance
            distance = d;
            location = i;
        end
    end
    
else
    
    if (location + window) > array_length
        %We need to wrap from the end
        % loop one - end of array:
        for i = (location-window):array_length
            d = (x-x_array(i))^2 + (y-y_array(i))^2;
            if d < distance
                distance = d;
                location = i;
            end
        end
        % loop two - start of array:
        for i = 1:(location+window-array_length)
            d = (x-x_array(i))^2 + (y-y_array(i))^2;
            if d < distance
                distance = d;
                location = i;
            end
        end
        
    elseif (location-window) < 1
        %We need to wrap from the beginning
        % loop one - end of array:
        for i = (array_length+location-window):array_length
            d = (x-x_array(i))^2 + (y-y_array(i))^2;
            if d < distance
                distance = d;
                location = i;
            end
        end
        % loop two - start of array:
        for i = 1:(location+window)
            d = (x-x_array(i))^2 + (y-y_array(i))^2;
            if d < distance
                distance = d;
                location = i;
            end
        end
        
    else
        %no need to wrap
        for i = (location-window):(location+window)
            d = (x-x_array(i))^2 + (y-y_array(i))^2;
            if d < distance
                distance = d;
                location = i;
            end
        end
    end
    
end
distance = sqrt(distance);
end

== matlab function QCar2_Virtual_Car2/Speed & Steering Commander/Path Commander/Path 6  Look Ahead Generator/Windowed Closest Point Locator *Feedback the location1 ==
  data: x input; location output; y input; x_array input; y_array input; window input; global_search input; distance output; previous_location input
function [location,distance] = find_closest_window_point(x,y,x_array,y_array, window, global_search, previous_location)
distance = 1e6;
location = previous_location;
array_length = length (x_array);

if (global_search == 1)
    
    %Search the whole array (usually at startup)
    for i =1:array_length
        d = (x-x_array(i))^2 + (y-y_array(i))^2;
        if d < distance
            distance = d;
            location = i;
        end
    end
    
else
    
    if (location + window) > array_length
        %We need to wrap from the end
        % loop one - end of array:
        for i = (location-window):array_length
            d = (x-x_array(i))^2 + (y-y_array(i))^2;
            if d < distance
                distance = d;
                location = i;
            end
        end
        % loop two - start of array:
        for i = 1:(location+window-array_length)
            d = (x-x_array(i))^2 + (y-y_array(i))^2;
            if d < distance
                distance = d;
                location = i;
            end
        end
        
    elseif (location-window) < 1
        %We need to wrap from the beginning
        % loop one - end of array:
        for i = (array_length+location-window):array_length
            d = (x-x_array(i))^2 + (y-y_array(i))^2;
            if d < distance
                distance = d;
                location = i;
            end
        end
        % loop two - start of array:
        for i = 1:(location+window)
            d = (x-x_array(i))^2 + (y-y_array(i))^2;
            if d < distance
                distance = d;
                location = i;
            end
        end
        
    else
        %no need to wrap
        for i = (location-window):(location+window)
            d = (x-x_array(i))^2 + (y-y_array(i))^2;
            if d < distance
                distance = d;
                location = i;
            end
        end
    end
    
end
distance = sqrt(distance);
end

== matlab function QCar2_Virtual_Car2/Infrastructure/Find Closest Car/MATLAB Function ==
  data: x_car input; distance output; y_car input; x_vector input; y_vector input; car_index input; heading input; proximity_radius input; proximity_scan_window input; max_distance input; distance_vector output; heading_vector output
function [distance, distance_vector, heading_vector] = proximity_sensor (x_car, y_car, x_vector, y_vector, car_index, heading, proximity_radius, proximity_scan_window, max_distance)
distance = max_distance;
distance_vector = max_distance*[1; 1; 1; 1; 1];
% heading_vector = 2*pi +  0*x_vector;
heading_vector = 2*pi*[1; 1; 1; 1; 1];

for i = 1:length (x_vector)
    if (i ~= car_index)
        distance_vector(i) = sqrt ((x_car - x_vector(i))^2 + (y_car - y_vector(i))^2);
        heading_vector(i) = atan2( (y_vector(i) - y_car), (x_vector(i) - x_car)) - heading;
        if (heading_vector(i) > pi)
            heading_vector(i) = heading_vector(i) - 2*pi;
        elseif (heading_vector(i) < -pi)
            heading_vector(i) = heading_vector(i) + 2*pi;
        end
        if ((distance_vector(i) < distance) && (abs (heading_vector(i)) <= proximity_scan_window))
            distance =  distance_vector(i);
        end
       
    end
end

== matlab function QCar2_Virtual_Car2/Infrastructure/Find Closest Car/MATLAB Function1 ==
  data: speed input; proximity_scan_window output; max_speed input; min_window input; max_window input
function proximity_scan_window = scan_window_generator(speed, max_speed, min_window, max_window)
%#codegen
proximity_scan_window = min_window + speed*(max_window - min_window) / max_speed;
end

== matlab function QCar2_Virtual_Car2/QCar/Virtual QCar/LED Logic/MATLAB Function ==
  data: headlights input; lights output; breaklights input; reverseLights input; leftTurn input; rightTurn input; pulse input
function lights = fcn (headlights, breaklights, reverseLights, leftTurn, rightTurn, pulse)

lights = zeros(1,16);
brakes = zeros(1,4); %4
head = zeros(1,6);%6
left = zeros(1,2);%2
right = zeros(1,2);%2
reverse = zeros(1,2);%2

if breaklights
    brakes = ones(1,4);
end

if headlights
    head = ones(1,6);
end

if reverseLights
    reverse = ones(1,2);
end

if leftTurn
    left = ones(1,2);
end

if rightTurn
    right = ones(1,2);
end

right = right & pulse;
left = left & pulse;

lights(1:4) = brakes;
lights(5:6) = reverse;
lights(7) = left(1);
lights(8) = right(1);
lights(9:14) = head;
lights(15) = left(2);
lights(16) = right(2);
